simulink model "labjede"  (R2021b)
settings: Solver=FixedStepAuto  StartTime=0.0  StopTime=10  FixedStep=0.01  RelTol=1e-3
settings Model: Creator=sucho  LastModifiedBy=sucho

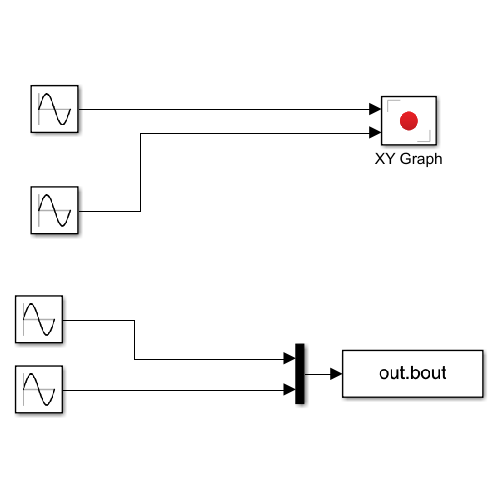
[thumbnail: Simulink's stored preview of the top-level diagram]
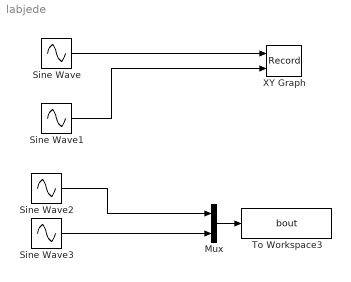
== system labjede ==
  Mux : Mux  Inputs=2
  Sine Wave : Sin  Amplitude=5  Frequency=5  Phase=pi/4  SampleTime=0
  Sine Wave1 : Sin  Frequency=3  SampleTime=0
  Sine Wave2 : Sin  Amplitude=5  Frequency=5  Phase=pi/4  SampleTime=0
  Sine Wave3 : Sin  Frequency=3  SampleTime=0
  To Workspace3 : ToWorkspace  VariableName=bout  SaveFormat=Timeseries  SampleTime=-1
      settings: Save2DSignal=2-D array (concatenate along first dimension)
  XY Graph : Record  FileSettingsInternal="{\"entries\":[{\"content\":{\"excelSettings\":{\"content\":{},\"type\":\"Streamout.ExcelSettings\"}},\"type\":\"Streamout.FileSettingStorage\",\"uuid\":\"d5bb5eab-9669-4695-a479-2f3820ce15dc\"}],\"packageUris\":[\"http://schema.mathworks.com/mf0/streamout_blocks/R2020a\"],\"version\":\"1.0\"}"  Layout=[1 1]  SignalsInternal="{\"entries\":[{\"content\":{\"signals\":[{\"content\":{\"blockPath\":[\"labjede/XY Graph\"],\"channel\":[],\"dimensions\":[1],\"domain\":\"labjede/XY Graph\",\"lineColor\":\"#a2142f\",\"plots\":[1],\"port\":1,\"sid\":[\"\"],\"signalID\":78,\"signalName\":\"Sine Wave\"},\"type\":\"RecordBlkView.Signal\",\"uuid\":\"ac937191-f08e-46cf-9135-0c9cf836cba0\"},{\"content\":{\"blockPath\":[\"labjede/XY Graph\"],\"channel\":[],\"dimensions\":[1],\"domain\":\"labjede/XY Graph\",\"lineColor\":\"#139fff\",\"plots\":[1],\"port\":2,\"sid\":[\"\"],\"signalID\":82,\"signalName\":\"Sine Wave1\"},\"type\":\"RecordBlkView.Signal\",\"uuid\":\"fe6ac4c3-211a-46df-a69c-e04f17881f0f\"}]},\"type\":\"RecordBlkView.InputSignals\",\"uuid\":\"a5c681ca-2213-496f-b78c-fd983f762260\"}],\"packageUris\":[\"http://schema.mathworks.com/mf0/streamout_blocks/R2020a\"],\"version\":\"1.0\"}"  VisualizationBindings="{\"xyplotplugin\":{\"info\":[{\"series\":[{\"bindingParametersList\":[{\"parameter\":\"X-Axis\",\"signalID\":78,\"signalName\":\"Sine Wave\"},{\"parameter\":\"Y-Axis\",\"signalID\":82,\"signalName\":\"Sine Wave1\"}],\"seriesID\":58539}],\"subplotID\":1}]}}"  CompatibilityTag=XY
  wires:
  Sine Wave/1 -> XY Graph/1
  Sine Wave1/1 -> XY Graph/2
  Sine Wave3/1 -> Mux/2
  Sine Wave2/1 -> Mux/1
  Mux/1 -> To Workspace3/1
